simulink model "movement_control_of_a_drone"  (R2022a)
settings: Solver=VariableStepAuto  StartTime=0.0  StopTime=5  RelTol=1e-3
(part 2 of 2)

== matlab function movement_control_of_a_drone/Pole 1 N pole ==
  data: u input; y output; c input
function y = voltage_control(u,c)

y = u*c;

end

== matlab function movement_control_of_a_drone/Pole 2 N pole ==
  data: u input; y output; c input
function y = voltage_control(u,c)

y = u*c;

end

== matlab function movement_control_of_a_drone/Pole 2 S pole ==
  data: u input; y output; c input
function y = voltage_control(u,c)

y = u*c;

end

== matlab function movement_control_of_a_drone/Pole 3 N pole ==
  data: u input; y output; c input
function y = voltage_control(u,c)

y = u*c;

end

== matlab function movement_control_of_a_drone/Pole 3 S pole ==
  data: u input; y output; c input
function y = voltage_control(u,c)

y = u*c;

end

== matlab function movement_control_of_a_drone/Pole 1 S pole ==
  data: u input; y output; c input
function y = voltage_control(u,c)

y = u*c;

end
